simulink model "IP_car"  (R2020b)
settings: Solver=VariableStepAuto  StartTime=0.0  StopTime=30  RelTol=1e-3
values from neighbouring files (symbols this model uses):
  g = 9.81    [Parameters.m]
  I = m*ell^2/12    [Parameters.m]
  l = 1    [Parameters.m]
  mc = 10    [Parameters.m]
  mp = 0.1    [Parameters.m]
libraries: pid_lib x1
settings Model: Creator=arthur  LastModifiedBy=arthur

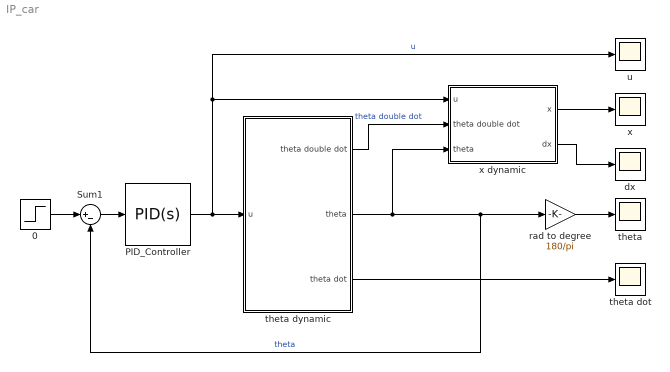
== system IP_car ==
  0 : Step  Time=0  After=0  SampleTime=0
  PID_Controller : pid_lib/PID Controller  Controller=PID  Form=Parallel  TimeDomain=Continuous-time  UseExternalTs=off  SampleTime=-1  IntegratorMethod=Forward Euler  FilterMethod=Forward Euler  ControllerParametersSource=internal  P=20  I=10  D=2  UseFilter=on  N=207.017575498237  TunerSelectOption=Transfer Function Based (PID Tuner App)  InitialConditionSource=internal  InitialConditionForIntegrator=0  InitialConditionForFilter=0  DifferentiatorICPrevScaledInput=0  ExternalReset=none  TrackingMode=off  Kt=1  LimitOutput=off  SatLimitsSource=internal  UpperSaturationLimit=inf  LowerSaturationLimit=-inf  LinearizeAsGain=on  AntiWindupMode=none  Kb=1  POutMin=[]  POutMax=[]  IOutMin=[]  IOutMax=[]  DOutMin=[]  DOutMax=[]  NOutMin=[]  NOutMax=[]  SumOutMin=[]  SumOutMax=[]  SaturationOutMin=[]  SaturationOutMax=[]  PParamMin=[]  PParamMax=[]  IParamMin=[]  IParamMax=[]  DParamMin=[]  DParamMax=[]  NParamMin=[]  NParamMax=[]  KbParamMin=[]  KbParamMax=[]  KtParamMin=[]  KtParamMax=[]  KbOutMin=[]  KbOutMax=[]  KtOutMin=[]  KtOutMax=[]  IntegratorOutMin=[]  IntegratorOutMax=[]  FilterOutMin=[]  FilterOutMax=[]  SumI1OutMin=[]  SumI1OutMax=[]  SumI2OutMin=[]  SumI2OutMax=[]  SumI3OutMin=[]  SumI3OutMax=[]  SumI4OutMin=[]  SumI4OutMax=[]  SumDOutMin=[]  SumDOutMax=[]  DifferentiatorOutMin=[]  DifferentiatorOutMax=[]  FilterDiffOutCoefMin=[]  FilterDiffOutCoefMax=[]  ReciprocalOutMin=[]  ReciprocalOutMax=[]  SumDenOutMin=[]  SumDenOutMax=[]  SumNumOutMin=[]  SumNumOutMax=[]  DivideOutMin=[]  DivideOutMax=[]  UdiffTsProdOutMin=[]  UdiffTsProdOutMax=[]  NTsProdOutMin=[]  NTsProdOutMax=[]  UintegralTsProdOutMin=[]  UintegralTsProdOutMax=[]  UngainTsProdOutMin=[]  UngainTsProdOutMax=[]  IntegratorContinuousStateAttributes=''  IntegratorStateMustResolveToSignalObject=off  IntegratorRTWStateStorageClass=Auto  FilterContinuousStateAttributes=''  FilterStateMustResolveToSignalObject=off  FilterRTWStateStorageClass=Auto  ParallelPVariant=InternalParameters  IdealPVariant=Disabled  IVariant=InternalParameters  DVariant=InternalParameters  IntegratorVariant=Continuous  SatVariant=Disabled  AWVariant=Passthrough  PCopyVariant=Disabled  TRVariant=Disabled  FdbkBlocksVariant=Forward  IdealPFdbkVariant=Disabled  SatFdbkVariant=Disabled  DerivativeFilterVariant=ContFilter  NVariant=InternalParameters  NCopyVariant=Disabled  FilterICVariant=InternalICsFilter  IntegratorICVariant=InternalICs  ExternalResetVariant=Disabled  TRSumVariant=Passthrough  SumFdbkVariant=Disabled  SumVariant=Sum_PID  TsampFilterVariant=InternalTs  TsampNgainVariant=Passthrough  TsampIntegralVariant=Passthrough  ExternalSaturationOutDataTypeStr=Inherit: Same as second input
  Sum1 : Sum  Inputs=|+-
  dx : Scope
  rad to degree : Gain  Gain=180/pi
  theta : Scope
  theta dot : Scope
  theta dynamic : Subsystem
  u : Scope
  x : Scope
  x dynamic : Subsystem
  wires:
  PID_Controller/1 -> u/1, x dynamic/1(u), theta dynamic/1(u)  "u"
  Sum1/1 -> PID_Controller/1
  0/1 -> Sum1/1
  theta dynamic/2(theta) -> rad to degree/1, Sum1/2, x dynamic/3(theta)  "theta"
  theta dynamic/1(theta double dot) -> x dynamic/2(theta double dot)  "theta double dot"
  x dynamic/1(x) -> x/1
  x dynamic/2(dx) -> dx/1
  rad to degree/1 -> theta/1
  theta dynamic/3(theta dot) -> theta dot/1

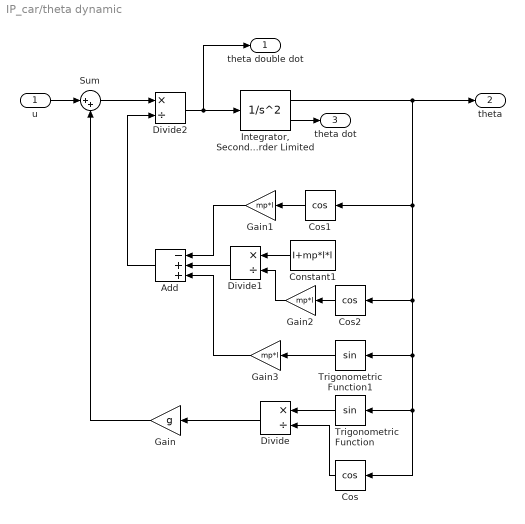
== system IP_car/theta dynamic ==
  u : Inport
  Add : Sum  Inputs=-++
  Constant1 : Constant  Value=I+mp*l*l
  Cos : Trigonometry  Operator=cos
  Cos1 : Trigonometry  Operator=cos
  Cos2 : Trigonometry  Operator=cos
  Divide : Product  Inputs=*/
  Divide1 : Product  Inputs=*/
  Divide2 : Product  Inputs=*/
  Gain : Gain  Gain=g
  Gain1 : Gain  Gain=mp*l
  Gain2 : Gain  Gain=mp*l
  Gain3 : Gain  Gain=mp*l
  "Integrator, Second-Order Limited" : SecondOrderIntegrator  ICX=1  LimitX=on  LimitDXDT=on
  Sum : Sum  Inputs=|++
  Trigonometric Function : Trigonometry
  Trigonometric Function1 : Trigonometry
  theta double dot : Outport
  theta : Outport  Port=2
  theta dot : Outport  Port=3
  wires:
  "Integrator, Second-Order Limited"/2 -> theta dot/1
  Gain/1 -> Sum/2
  Trigonometric Function/1 -> Divide/1
  Gain3/1 -> Add/3
  Cos2/1 -> Gain2/1
  Divide1/1 -> Add/2
  Gain2/1 -> Divide1/2
  Divide2/1 -> theta double dot/1, "Integrator, Second-Order Limited"/1
  u/1 -> Sum/1
  Cos1/1 -> Gain1/1
  Add/1 -> Divide2/2
  Sum/1 -> Divide2/1
  Trigonometric Function1/1 -> Gain3/1
  Divide/1 -> Gain/1
  Gain1/1 -> Add/1
  Constant1/1 -> Divide1/1
  Cos/1 -> Divide/2
  "Integrator, Second-Order Limited"/1 -> theta/1, Cos1/1, Cos/1, Trigonometric Function/1, Trigonometric Function1/1, Cos2/1

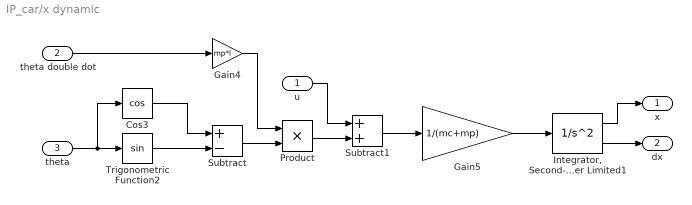
== system IP_car/x dynamic ==
  u : Inport
  theta double dot : Inport  Port=2
  theta : Inport  Port=3
  Cos3 : Trigonometry  Operator=cos
  Gain4 : Gain  Gain=mp*l
  Gain5 : Gain  Gain=1/(mc+mp)
  "Integrator, Second-Order Limited1" : SecondOrderIntegrator  ICX=0  LimitX=on  LimitDXDT=on
  Product : Product
  Subtract : Sum  Inputs=+-
  Subtract1 : Sum
  Trigonometric Function2 : Trigonometry
  x : Outport
  dx : Outport  Port=2
  wires:
  theta/1 -> Trigonometric Function2/1, Cos3/1
  Subtract1/1 -> Gain5/1
  Subtract/1 -> Product/2
  Trigonometric Function2/1 -> Subtract/2
  "Integrator, Second-Order Limited1"/1 -> x/1
  theta double dot/1 -> Gain4/1
  Gain4/1 -> Product/1
  u/1 -> Subtract1/1
  Cos3/1 -> Subtract/1
  Product/1 -> Subtract1/2
  Gain5/1 -> "Integrator, Second-Order Limited1"/1
  "Integrator, Second-Order Limited1"/2 -> dx/1
